simulink model "sim_2026_cart_pend"  (R2025b)
settings: Solver=ode45  StartTime=0.0  StopTime=10  MinStep=0.5*ts  RelTol=1e-3
values from neighbouring files (symbols this model uses):
  alpha_o = 0    [main_Q33_Q34.m]
  bc = (M + m) * b_hat    [main_Q33_Q34.m]
  bp = m * (lp^2) * a_hat1    (= 0.003770779032)    [main_Q33_Q34.m]
  g = 9.81    [main_Q33_Q34.m]
  Kv = (M + m) * a_hat    [main_Q33_Q34.m]
  lp = g / a_hat0    (= 0.254276827372)    [main_Q33_Q34.m]
  m = 0.1    [main_Q33_Q34.m]
  ts = 0.002    [data_TFs_cart_pend.mat]    (also in data_test_01.mat; data_test_67.mat)
  vc_o = 0    [main_Q33_Q34.m]
  w_o = 0    [main_Q33_Q34.m]
  xc_o = 0    [main_Q33_Q34.m]
undefined symbols (not defined in the file or in its folder): M
libraries: simulink x1
settings Model: Creator=ricardoaguilera  LastModifiedBy=jaylen
settings SolverCC: AlgebraicLoopSolver=TrustRegion
settings DataIOCC: ReturnWorkspaceOutputs=off
settings OptimizationCC: LifeSpan=inf
settings DebuggingCC: UnconnectedInputMsg=warning  UnconnectedOutputMsg=warning  UnconnectedLineMsg=warning  ArithmeticOperatorsInVariantConditions=warning
settings ModelReferenceCC: EnableRefExpFcnMdlSchedulingChecks=on
settings SFSimCC: CustomCodeUndefinedFunction=UseInterfaceOnly
settings RTWCC: GPUComputeCapability=3.5  DLArmComputeVersion=19.05
settings CodeAppCC: StateflowObjectComments=on

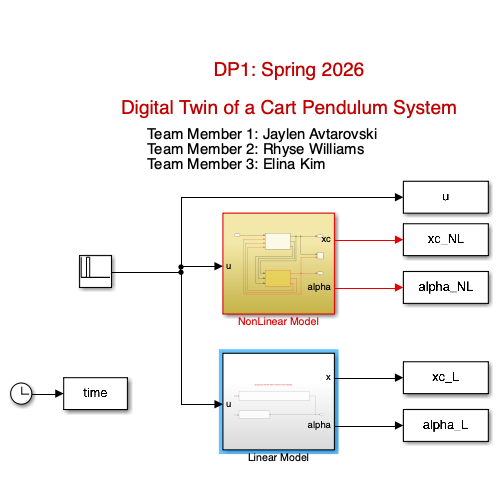
[thumbnail: Simulink's stored preview of the top-level diagram]
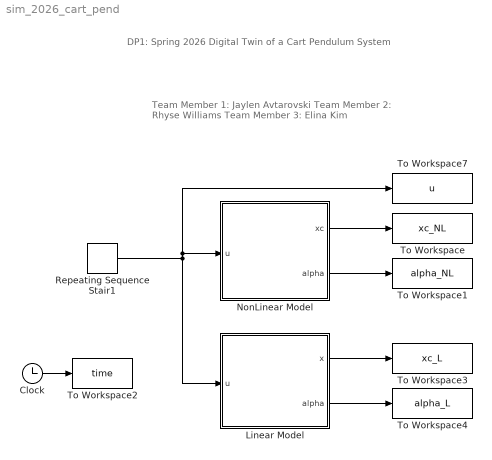
== system sim_2026_cart_pend ==
  note: DP1: Spring 2026
      |
      | Digital Twin of a Cart Pendulum System
  note: Team Member 1: Jaylen Avtarovski
      | Team Member 2: Rhyse Williams
      | Team Member 3: Elina Kim
  Clock : Clock
  Linear Model : Subsystem
  NonLinear Model : Subsystem
  Repeating Sequence Stair1 : simulink/Sources/Repeating Sequence Stair  OutValues=[0 0 4 0 0 0 0 0 0 0].'  tsamp=1  OutMin=[]  OutMax=[]  OutDataTypeStr=double  OutputDataTypeScalingMode=double  OutDataType=fixdt(0,8)  ConRadixGroup=Best Precision: Vector-wise  OutScaling=2^-12
  To Workspace : ToWorkspace  VariableName=xc_NL  SampleTime=ts
  To Workspace1 : ToWorkspace  VariableName=alpha_NL  SampleTime=ts
  To Workspace2 : ToWorkspace  VariableName=time  SampleTime=ts
  To Workspace3 : ToWorkspace  VariableName=xc_L  SampleTime=ts
  To Workspace4 : ToWorkspace  VariableName=alpha_L  SampleTime=ts
  To Workspace7 : ToWorkspace  VariableName=u  SampleTime=ts
  wires:
  Clock/1 -> To Workspace2/1
  NonLinear Model/1(xc) -> To Workspace/1
  NonLinear Model/2(alpha) -> To Workspace1/1
  Linear Model/1(x) -> To Workspace3/1
  Linear Model/2(alpha) -> To Workspace4/1
  Repeating Sequence Stair1/1 -> To Workspace7/1, NonLinear Model/1(u), Linear Model/1(u)

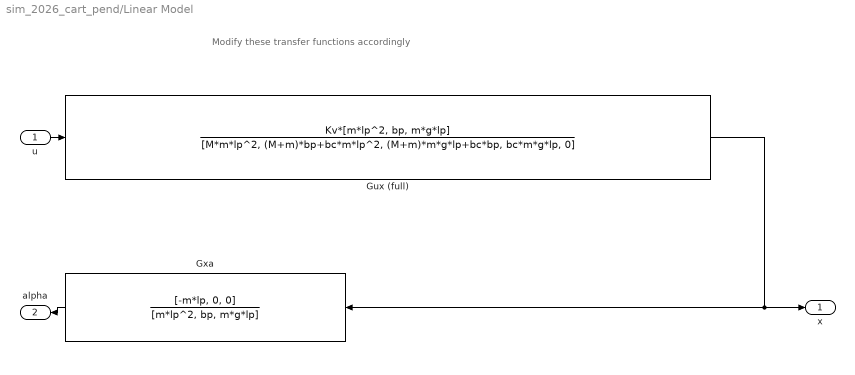
== system sim_2026_cart_pend/Linear Model ==
  note: Modify these transfer functions accordingly
  u : Inport
  Gux (full) : TransferFcn  Numerator=Kv*[m*lp^2, bp, m*g*lp]  Denominator=[M*m*lp^2, (M+m)*bp+bc*m*lp^2, (M+m)*m*g*lp+bc*bp, bc*m*g*lp, 0]
  Gxa : TransferFcn  Numerator=[-m*lp, 0, 0]  Denominator=[m*lp^2, bp, m*g*lp]
  x : Outport  VectorParamsAs1DForOutWhenUnconnected=off
  alpha : Outport  Port=2  VectorParamsAs1DForOutWhenUnconnected=off
  wires:
  Gux (full)/1 -> Gxa/1, x/1
  u/1 -> Gux (full)/1
  Gxa/1 -> alpha/1

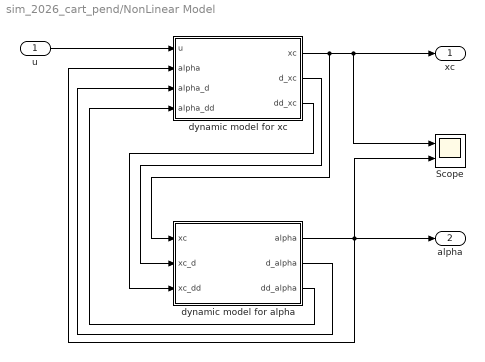
== system sim_2026_cart_pend/NonLinear Model ==
  u : Inport
  Scope : Scope  NumInputPorts=2
      settings: ActiveDisplayYMinimum=-0.5052  ActiveDisplayYMaximum=4.54678
  dynamic model for alpha : Subsystem
  dynamic model for xc : Subsystem
  xc : Outport  VectorParamsAs1DForOutWhenUnconnected=off
  alpha : Outport  Port=2  VectorParamsAs1DForOutWhenUnconnected=off
  wires:
  dynamic model for alpha/3(dd_alpha) -> dynamic model for xc/4(alpha_dd)
  dynamic model for xc/1(xc) -> dynamic model for alpha/1("xc "), xc/1, Scope/1
  u/1 -> dynamic model for xc/1(u)
  dynamic model for alpha/2(d_alpha) -> dynamic model for xc/3(alpha_d)
  dynamic model for xc/3(dd_xc) -> dynamic model for alpha/3(xc_dd)
  dynamic model for alpha/1(alpha) -> Scope/2, alpha/1, dynamic model for xc/2(alpha)
  dynamic model for xc/2(d_xc) -> dynamic model for alpha/2(xc_d)

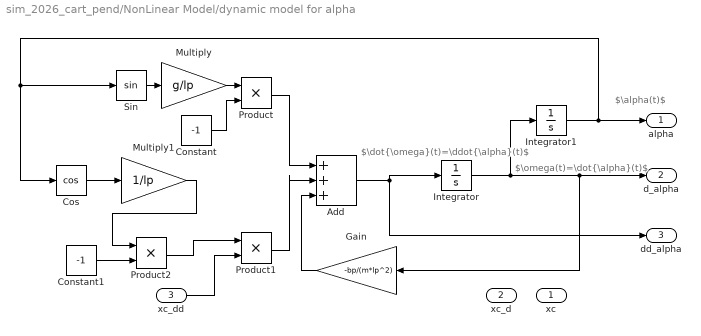
== system sim_2026_cart_pend/NonLinear Model/dynamic model for alpha ==
  note: $\dot{\omega}(t)=\ddot{\alpha}(t)$
  note: $\omega(t)=\dot{\alpha}(t)$
  note: $\alpha(t)$
  "xc " : Inport
  xc_d : Inport  Port=2
  xc_dd : Inport  Port=3
  Add : Sum  Inputs=++|+
  Constant : Constant  Value=-1
  Constant1 : Constant  Value=-1
  Cos : Trigonometry  Operator=cos
  Gain : Gain  Gain=-bp/(m*lp^2)
  Integrator : Integrator  InitialCondition=w_o
  Integrator1 : Integrator  InitialCondition=alpha_o
  Multiply : Gain  Gain=g/lp
  Multiply1 : Gain  Gain=1/lp
  Product : Product
  Product1 : Product
  Product2 : Product
  Sin : Trigonometry
  alpha : Outport  VectorParamsAs1DForOutWhenUnconnected=off
  d_alpha : Outport  Port=2  VectorParamsAs1DForOutWhenUnconnected=off
  dd_alpha : Outport  Port=3  VectorParamsAs1DForOutWhenUnconnected=off
  wires:
  Integrator1/1 -> Sin/1, Cos/1, alpha/1
  Integrator/1 -> Gain/1, d_alpha/1, Integrator1/1
  Cos/1 -> Multiply1/1
  Multiply1/1 -> Product2/1
  Product2/1 -> Product1/1
  xc_dd/1 -> Product1/2
  Multiply/1 -> Product/1
  Product1/1 -> Add/2
  Product/1 -> Add/1
  Constant/1 -> Product/2
  Add/1 -> Integrator/1, dd_alpha/1
  Constant1/1 -> Product2/2
  Sin/1 -> Multiply/1
  Gain/1 -> Add/3

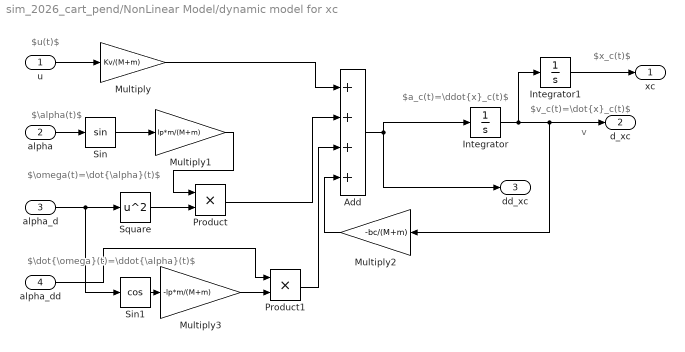
== system sim_2026_cart_pend/NonLinear Model/dynamic model for xc ==
  note: $x_c(t)$
  note: v
  note: $v_c(t)=\dot{x}_c(t)$
  note: $a_c(t)=\ddot{x}_c(t)$
  note: $\alpha(t)$
  note: $\omega(t)=\dot{\alpha}(t)$
  note: $\dot{\omega}(t)=\ddot{\alpha}(t)$
  note: $u(t)$
  u : Inport
  alpha : Inport  Port=2
  alpha_d : Inport  Port=3
  alpha_dd : Inport  Port=4
  Add : Sum  Inputs=++++
  Integrator : Integrator  InitialCondition=vc_o
  Integrator1 : Integrator  InitialCondition=xc_o
  Multiply : Gain  Gain=Kv/(M+m)
  Multiply1 : Gain  Gain=lp*m/(M+m)
  Multiply2 : Gain  Gain=-bc/(M+m)
  Multiply3 : Gain  Gain=-lp*m/(M+m)
  Product : Product
  Product1 : Product
  Sin : Trigonometry
  Sin1 : Trigonometry  Operator=cos
  Square : Math  Operator=square
  xc : Outport  VectorParamsAs1DForOutWhenUnconnected=off
  d_xc : Outport  Port=2  VectorParamsAs1DForOutWhenUnconnected=off
  dd_xc : Outport  Port=3  VectorParamsAs1DForOutWhenUnconnected=off
  wires:
  Add/1 -> dd_xc/1, Integrator/1
  Integrator1/1 -> xc/1
  Integrator/1 -> d_xc/1, Multiply2/1, Integrator1/1
  Multiply2/1 -> Add/4
  alpha/1 -> Sin/1
  Sin1/1 -> Multiply3/1
  Multiply/1 -> Add/1
  alpha_dd/1 -> Product1/1
  Sin/1 -> Multiply1/1
  Product1/1 -> Add/3
  Square/1 -> Product/2
  Multiply3/1 -> Product1/2
  Multiply1/1 -> Product/1
  Product/1 -> Add/2
  alpha_d/1 -> Sin1/1, Square/1
  u/1 -> Multiply/1
